simulink library "Lib_Piccolo"  (R2018b)
settings: Solver=VariableStepAuto  StartTime=0.0  StopTime=10.0  RelTol=1e-3
values from neighbouring files (symbols this model uses):
  AccelErrInt2Brakes = 0.15    [SimulationControlConfig16P.m]    (also in SimulationControlConfig16P_F0.m; SimulationControlConfig16P_F2.m; SimulationControlConfig16P_LEGACY.m; SimulationControlConfigTAILLESS.m = 0.2)
  AileronMax = 25    [SimulationControlConfig16P.m]    (also in SimulationControlConfig16P_F0.m; SimulationControlConfig16P_F2.m; SimulationControlConfig16P_LEGACY.m; SimulationControlConfigTAILLESS.m)
  AileronPower = 0.00268    [SimulationControlConfig16P.m]    (also in SimulationControlConfig16P_F0.m; SimulationControlConfig16P_F2.m; SimulationControlConfig16P_LEGACY.m; SimulationControlConfigTAILLESS.m = 0.002266)
  AileronSurfaceMax = 45    [SimulationControlConfig16P.m]    (also in SimulationControlConfig16P_F0.m; SimulationControlConfig16P_F2.m; SimulationControlConfig16P_LEGACY.m; SimulationControlConfigTAILLESS_CGAFT_F0.m = 25)
  AileronTrim = 0    [SimulationControlConfig16P.m]    (also in SimulationControlConfig16P_F0.m; SimulationControlConfig16P_F2.m; SimulationControlConfig16P_LEGACY.m; SimulationControlConfigTAILLESS.m)
  Alt = 1000 + TerrainHeight    [SimulationStateConfig.m]
  AltCruise_m = Alt * 0.3048    [SimulationControlConfig16P.m]    (also in SimulationControlConfig16P_F2.m; SimulationControlConfigTAILLESS.m = Alt/3.28084; SimulationControlConfigTAILLESS_CGAFT_F0.m = 640; SimulationControlConfigTAILLESS_CGFWD_F0.m = 640)
  AltitudeRate2PitchCmdIntegratorInit = 0.1    [SimulationControlPre.m]
  AltMax = 10000    [SimulationControlConfig16P.m]    (also in SimulationControlConfig16P_F0.m; SimulationControlConfig16P_F2.m; SimulationControlConfig16P_LEGACY.m; SimulationControlConfigTAILLESS.m)
  AltMaxAccel = 2.5    [SimulationControlConfig16P.m]    (also in SimulationControlConfig16P_F0.m = 2; SimulationControlConfig16P_F2.m = 2; SimulationControlConfig16P_LEGACY.m = 0.9; SimulationControlConfigTAILLESS.m = 2)
  AltMin = 0    [SimulationControlConfig16P.m]    (also in SimulationControlConfig16P_F0.m; SimulationControlConfig16P_F2.m; SimulationControlConfig16P_LEGACY.m; SimulationControlConfigTAILLESS.m)
  AltRateCmd2Pitch = 0.26    [SimulationControlConfig16P.m]    (also in SimulationControlConfig16P_F0.m = 0.35; SimulationControlConfig16P_F2.m = 0.35; SimulationControlConfig16P_LEGACY.m = 0.6; SimulationControlConfigTAILLESS.m = 0.9)
  AltRateError2Pitch = 0.34    [SimulationControlConfig16P.m]    (also in SimulationControlConfig16P_F0.m = 0.61; SimulationControlConfig16P_F2.m = 0.61; SimulationControlConfig16P_LEGACY.m = 0.4; SimulationControlConfigTAILLESS.m = 0.3)
  AltRateErrorInt2Pitch = 0.61    [SimulationControlConfig16P.m]    (also in SimulationControlConfig16P_F0.m = 0.28; SimulationControlConfig16P_F2.m = 0.28; SimulationControlConfig16P_LEGACY.m = 0.45; SimulationControlConfigTAILLESS.m = 0.15)
  AltRateLpfCutOff = 3    [SimulationControlConfig16P.m]    (also in SimulationControlConfig16P_F0.m; SimulationControlConfig16P_F2.m; SimulationControlConfig16P_LEGACY.m; SimulationControlConfigTAILLESS.m = 5)
  AutoNosegear2Rudder = 26    [SimulationControlConfig16P.m]    (also in SimulationControlConfig16P_F0.m; SimulationControlConfig16P_F2.m; SimulationControlConfig16P_LEGACY.m; SimulationControlConfigTAILLESS.m = 25.2)
  b = 5.54    [SimulationControlConfig16P.m]    (also in SimulationControlConfig16P_F0.m; SimulationControlConfig16P_F2.m; SimulationControlConfig16P_LEGACY.m; SimulationControlConfigTAILLESS.m = 2.37)
  Bank2AileronIntegratorInit = 0    [SimulationControlPre.m]
  BankMax_User = BankMax_User/180*pi    (= 0.610865238198)    [SimulationControlConfig16P.m]    (also in SimulationControlConfig16P_F0.m = 0.523598775598; SimulationControlConfig16P_F2.m = 0.523598775598; SimulationControlConfig16P_LEGACY.m = 0.523598775598; SimulationControlConfigTAILLESS.m = 0.558505360638)
  baseLegFlaps = 20    [SimulationControlConfig16P.m]    (also in SimulationControlConfig16P_F0.m; SimulationControlConfig16P_F2.m = 15; SimulationControlConfig16P_LEGACY.m = 0; SimulationControlConfigTAILLESS.m = 0)
  C = GeneticOpt.C    [SimulationCostFunction.m]
  c = Sw/b    (= 0.841696750903)    [SimulationControlConfig16P.m]    (also in SimulationControlConfig16P_F0.m; SimulationControlConfig16P_F2.m; SimulationControlConfig16P_LEGACY.m; SimulationControlConfigTAILLESS.m = 0.354008438819)
  cell2WheelFactorMG = 5.98    [SimulationSensorConfig16P_LEGACY.m]
  cell2WheelFactorNG = 1    [SimulationSensorConfig16P_LEGACY.m]
  cellSatMaxMG = 15000    [SimulationSensorConfig16P.m]    (also in SimulationSensorConfig16P_LEGACY.m; SimulationSensorConfigTAILLESS7P.m; SimulationSensorConfigUTAIL7P.m)
  cellSatMaxNG = 1000    [SimulationSensorConfig16P.m]    (also in SimulationSensorConfig16P_LEGACY.m; SimulationSensorConfigTAILLESS7P.m; SimulationSensorConfigUTAIL7P.m)
  cellSatMinMG = -15000    [SimulationSensorConfig16P.m]    (also in SimulationSensorConfig16P_LEGACY.m; SimulationSensorConfigTAILLESS7P.m; SimulationSensorConfigUTAIL7P.m)
  cellSatMinNG = -1000    [SimulationSensorConfig16P.m]    (also in SimulationSensorConfig16P_LEGACY.m; SimulationSensorConfigTAILLESS7P.m; SimulationSensorConfigUTAIL7P.m)
  CL_Limit = CL_Max    (= 0.54)    [SimulationControlConfig16P.m]    (also in SimulationControlConfig16P_F0.m; SimulationControlConfig16P_F2.m = 0.638; SimulationControlConfig16P_LEGACY.m; SimulationControlConfigTAILLESS.m = 0.525)
  CL_Max = 0.54    [SimulationControlConfig16P.m]    (also in SimulationControlConfig16P_F0.m; SimulationControlConfig16P_F2.m = 0.638; SimulationControlConfig16P_LEGACY.m; SimulationControlConfigTAILLESS.m = 0.525)
  CL_Max_Nom = 0.465    [SimulationControlConfig16P.m]    (also in SimulationControlConfig16P_F0.m; SimulationControlConfig16P_F2.m = 0.563; SimulationControlConfig16P_LEGACY.m; SimulationControlConfigTAILLESS.m = 0.39)
  CL_Min = 0    [SimulationControlConfig16P.m]    (also in SimulationControlConfig16P_F0.m; SimulationControlConfig16P_F2.m; SimulationControlConfig16P_LEGACY.m; SimulationControlConfigTAILLESS.m)
  ClimbMaxFraction = 0.35    [SimulationControlConfig16P.m]    (also in SimulationControlConfig16P_F0.m = 0.17; SimulationControlConfig16P_F2.m = 0.17; SimulationControlConfig16P_LEGACY.m = 0.24; SimulationControlConfigTAILLESS.m = 0.21)
  ClimboutMaxBank = 7.0    (= 7)    [SimulationControlConfig16P.m]    (also in SimulationControlConfig16P_F0.m; SimulationControlConfig16P_F2.m; SimulationControlConfig16P_LEGACY.m; SimulationControlConfigTAILLESS.m = 5)
  ClimboutTimer = 7.0    (= 7)    [SimulationControlConfig16P.m]    (also in SimulationControlConfig16P_F0.m; SimulationControlConfig16P_F2.m; SimulationControlConfig16P_LEGACY.m; SimulationControlConfigTAILLESS.m)
  dCl_per_dFlap = 0.005581818    [SimulationControlConfig16P.m]    (also in SimulationControlConfig16P_F0.m = 0; SimulationControlConfig16P_F2.m = 0.0065; SimulationControlConfig16P_LEGACY.m = 0; SimulationControlConfigTAILLESS.m = 0)
  DecelerationCmd = 3.1    [SimulationControlConfig16P.m]    (also in SimulationControlConfig16P_F0.m; SimulationControlConfig16P_F2.m; SimulationControlConfig16P_LEGACY.m; SimulationControlConfigTAILLESS.m = 0.1)
  DeRotateLogicEndTimer = abs((NoseDownLimit_Deg-1)/DeRotateRamp_Dps)    [SimulationControlConfig16P.m]    (also in SimulationControlConfig16P_F0.m; SimulationControlConfig16P_F2.m; SimulationControlConfig16P_LEGACY.m; SimulationControlConfigTAILLESS.m)
  DeRotateLogicHoldNoseUpTimer = 0.1    [SimulationControlConfig16P.m]    (also in SimulationControlConfig16P_F0.m; SimulationControlConfig16P_F2.m; SimulationControlConfig16P_LEGACY.m; SimulationControlConfigTAILLESS.m)
  DeRotateLogicTimerTimeout = 2    [SimulationControlConfig16P.m]    (also in SimulationControlConfig16P_F0.m; SimulationControlConfig16P_F2.m; SimulationControlConfig16P_LEGACY.m; SimulationControlConfigTAILLESS.m)
  DeRotateLowerCmdSaturation = 0    [SimulationControlConfig16P.m]    (also in SimulationControlConfig16P_F0.m; SimulationControlConfig16P_F2.m; SimulationControlConfig16P_LEGACY.m; SimulationControlConfigTAILLESS.m)
  DeRotateRamp_Dps = 3    [SimulationControlConfig16P.m]    (also in SimulationControlConfig16P_F0.m; SimulationControlConfig16P_F2.m; SimulationControlConfig16P_LEGACY.m; SimulationControlConfigTAILLESS.m = 8)
  DeRotateUpperCmdSaturation = 7    [SimulationControlConfig16P.m]    (also in SimulationControlConfig16P_F0.m; SimulationControlConfig16P_F2.m; SimulationControlConfig16P_LEGACY.m; SimulationControlConfigTAILLESS.m)
  DescentMaxFraction = 0.22    [SimulationControlConfig16P.m]    (also in SimulationControlConfig16P_F0.m = 0.2; SimulationControlConfig16P_F2.m = 0.2; SimulationControlConfig16P_LEGACY.m = 0.2; SimulationControlConfigTAILLESS.m = 0.17)
  DesktopSimTerrainOffset_m = 0.406    [SimulationAircraftConfig.m]
  downwindFlaps = 0    [SimulationControlConfig16P.m]    (also in SimulationControlConfig16P_F0.m; SimulationControlConfig16P_F2.m = 15; SimulationControlConfig16P_LEGACY.m; SimulationControlConfigTAILLESS.m)
  downwindSplitAil = 0    [SimulationControlConfig16P_F2.m]
  DP_init = 0.5*1.225*V_init^2    [SimulationControlConfig16P.m]    (also in SimulationControlConfig16P_F0.m; SimulationControlConfig16P_F2.m; SimulationControlConfig16P_LEGACY.m; SimulationControlConfigTAILLESS.m)
  dscNoiseMG = 1    [SimulationSensorConfig16P_LEGACY.m]
  dscNoiseNG = 0.25    [SimulationSensorConfig16P_LEGACY.m]
  DSCnumBits = 24    [SimulationSensorConfig16P.m]    (also in SimulationSensorConfig16P_LEGACY.m; SimulationSensorConfigTAILLESS7P.m; SimulationSensorConfigUTAIL7P.m)
  DSCRangeMaxMG = 15000    [SimulationSensorConfig16P.m]    (also in SimulationSensorConfig16P_LEGACY.m; SimulationSensorConfigTAILLESS7P.m; SimulationSensorConfigUTAIL7P.m)
  DSCRangeMaxNG = 1000    [SimulationSensorConfig16P.m]    (also in SimulationSensorConfig16P_LEGACY.m; SimulationSensorConfigTAILLESS7P.m; SimulationSensorConfigUTAIL7P.m)
  DSCRangeMinMG = -15000    [SimulationSensorConfig16P.m]    (also in SimulationSensorConfig16P_LEGACY.m; SimulationSensorConfigTAILLESS7P.m; SimulationSensorConfigUTAIL7P.m)
  DSCRangeMinNG = -1000    [SimulationSensorConfig16P.m]    (also in SimulationSensorConfig16P_LEGACY.m; SimulationSensorConfigTAILLESS7P.m; SimulationSensorConfigUTAIL7P.m)
  dt = DLLSim.dt    [SimulationTimeStep.m]    (also in SimulationTrim.m = 0.02)
  EarlyTouchdownThreshold = 3.0    (= 3)    [SimulationControlConfig16P.m]    (also in SimulationControlConfig16P_F0.m; SimulationControlConfig16P_F2.m; SimulationControlConfig16P_LEGACY.m; SimulationControlConfigTAILLESS.m)
  ElevatorDeflectionRate = 15    [SimulationControlConfig16P.m]    (also in SimulationControlConfig16P_F0.m; SimulationControlConfig16P_F2.m; SimulationControlConfig16P_LEGACY.m = 12; SimulationControlConfigTAILLESS.m = 5)
  ElevatorMax = 25    [SimulationControlConfig16P.m]    (also in SimulationControlConfig16P_F0.m; SimulationControlConfig16P_F2.m; SimulationControlConfig16P_LEGACY.m; SimulationControlConfigTAILLESS.m)
  ElevatorPower = -0.002209    [SimulationControlConfig16P.m]    (also in SimulationControlConfig16P_F0.m; SimulationControlConfig16P_F2.m; SimulationControlConfig16P_LEGACY.m; SimulationControlConfigTAILLESS.m = -0.002668)
  ElevatorTrim = -3.5    [SimulationControlConfig16P.m]    (also in SimulationControlConfig16P_F0.m; SimulationControlConfig16P_F2.m; SimulationControlConfig16P_LEGACY.m; SimulationControlConfigTAILLESS.m = -3)
  elevonBias = 0    [SimulationControlConfig16P.m]    (also in SimulationControlConfig16P_F0.m; SimulationControlConfig16P_F2.m; SimulationControlConfig16P_LEGACY.m; SimulationControlConfigTAILLESS.m)
  Enable_TAS_Protection = 0    [SimulationControlConfig16P.m]    (also in SimulationControlConfig16P_F0.m; SimulationControlConfig16P_F2.m; SimulationControlConfig16P_LEGACY.m; SimulationControlConfigTAILLESS.m)
  EnableCrossTrackAbort = 1    [SimulationControlConfig16P.m]    (also in SimulationControlConfigTAILLESS.m; SimulationControlConfigTAILLESS_CGAFT_F0.m; SimulationControlConfigTAILLESS_CGFWD_F0.m; SimulationControlConfigTAILLESS_CGFWD_F2.m)
  EnergyBandwidth = 0.04    [SimulationControlConfig16P.m]    (also in SimulationControlConfig16P_F0.m = 0.03; SimulationControlConfig16P_F2.m = 0.03; SimulationControlConfig16P_LEGACY.m = 0.02; SimulationControlConfigTAILLESS.m = 0.06)
  EngineLhFuelCut = 0    [SimulationAircraftConfig.m]
  EngineRhFuelCut = 0    [SimulationAircraftConfig.m]
  FastThrottleRate = 0.075    [SimulationControlConfig16P.m]    (also in SimulationControlConfig16P_F0.m = 0.05; SimulationControlConfig16P_F2.m = 0.05; SimulationControlConfig16P_LEGACY.m = 0.05; SimulationControlConfigTAILLESS.m = 0.1)
  FilterWarmUpTime = 2    [SimulationSensorConfig16P.m]    (also in SimulationSensorConfig16P_LEGACY.m; SimulationSensorConfigTAILLESS7P.m; SimulationSensorConfigUTAIL7P.m)
  finalApproachFlaps = 20    [SimulationControlConfig16P.m]    (also in SimulationControlConfig16P_F0.m; SimulationControlConfig16P_F2.m = 15; SimulationControlConfig16P_LEGACY.m = 0; SimulationControlConfigTAILLESS.m = 0)
  finalApproachSplitAil = 20    [SimulationControlConfig16P_F2.m]
  FinalDescentSlope_Deg = testPlans(testIndx).descentSlope    [SimulationControlConfig16P.m]    (also in SimulationControlConfig16P_F0.m; SimulationControlConfig16P_F2.m; SimulationControlConfig16P_LEGACY.m; SimulationControlConfigTAILLESS.m)
  flapMax = 0    [SimulationControlConfig16P.m]    (also in SimulationControlConfig16P_F0.m = 35; SimulationControlConfig16P_F2.m = 33; SimulationControlConfig16P_LEGACY.m; SimulationControlConfigTAILLESS.m)
  flapRate = 7.5    [SimulationControlConfig16P.m]    (also in SimulationControlConfig16P_F0.m; SimulationControlConfig16P_F2.m; SimulationControlConfig16P_LEGACY.m; SimulationControlConfigTAILLESS.m = 6.6)
  FlareHeight = 5    [SimulationControlConfig16P.m]    (also in SimulationControlConfig16P_F0.m; SimulationControlConfig16P_F2.m; SimulationControlConfig16P_LEGACY.m = 4.8; SimulationControlConfigTAILLESS.m = 2.75)
  FlareVerticalRate_mps = -0.4    [SimulationControlConfig16P.m]    (also in SimulationControlConfig16P_F0.m; SimulationControlConfig16P_F2.m; SimulationControlConfig16P_LEGACY.m = -0.5; SimulationControlConfigTAILLESS.m = -0.15)
  Fp_Aileron = 0.55*2*pi*RollRateLpfCutoff*dt    [SimulationControlConfig16P.m]    (also in SimulationControlConfig16P_F0.m; SimulationControlConfig16P_F2.m; SimulationControlConfig16P_LEGACY.m; SimulationControlConfigTAILLESS.m)
  Fp_Alt = 2*pi*0.55*AltBandwidth    (= 0.622035345411)    [SimulationControlConfig16P.m]    (also in SimulationControlConfig16P_F0.m; SimulationControlConfig16P_F2.m; SimulationControlConfig16P_LEGACY.m = 0.099; SimulationControlConfigTAILLESS.m = 0.207345115137)
  Fp_AltRate = 0.55*2*pi*AltRateLpfCutOff*dt    [SimulationControlConfig16P.m]    (also in SimulationControlConfig16P_F0.m; SimulationControlConfig16P_F2.m; SimulationControlConfig16P_LEGACY.m; SimulationControlConfigTAILLESS.m)
  Fp_Elevator = 0.55*2*pi*PitchRateLpfCutoff*dt    [SimulationControlConfig16P.m]    (also in SimulationControlConfig16P_F0.m; SimulationControlConfig16P_F2.m; SimulationControlConfig16P_LEGACY.m; SimulationControlConfigTAILLESS.m)
  Fp_Energy = 0.55*2*pi*EnergyBandwidth    (= 0.138230076758)    [SimulationControlConfig16P.m]    (also in SimulationControlConfig16P_F0.m = 0.103672557568; SimulationControlConfig16P_F2.m = 0.103672557568; SimulationControlConfig16P_LEGACY.m = 0.069115038379; SimulationControlConfigTAILLESS.m = 0.207345115137)
  Fp_Energy2 = 0.55*2*pi*EnergyBandwidth*dt    [SimulationControlConfig16P.m]    (also in SimulationControlConfig16P_F0.m; SimulationControlConfig16P_F2.m; SimulationControlConfig16P_LEGACY.m; SimulationControlConfigTAILLESS.m)
  Fp_Pitch = 0.55*2*pi*PitchBandwidth    (= 2.45358386245)    [SimulationControlConfig16P.m]    (also in SimulationControlConfig16P_F0.m; SimulationControlConfig16P_F2.m = 1.72787595947; SimulationControlConfig16P_LEGACY.m = 3.11017672705; SimulationControlConfigTAILLESS.m = 1.55508836353)
  Fp_Pitch_2 = 0.55*2*pi*PitchBandwidth*dt    [SimulationControlConfig16P.m]    (also in SimulationControlConfig16P_F0.m; SimulationControlConfig16P_F2.m; SimulationControlConfig16P_LEGACY.m; SimulationControlConfigTAILLESS.m)
  Fp_Roll = RollBandwidth^2    (= 1.69)    [SimulationControlConfig16P.m]    (also in SimulationControlConfig16P_F0.m = 1.44; SimulationControlConfig16P_F2.m = 1.44; SimulationControlConfig16P_LEGACY.m = 1.44; SimulationControlConfigTAILLESS.m = 1.21)
  Fp_Rudder = 0.55*2*pi*YawRateLpfCutoff*dt    [SimulationControlConfig16P.m]    (also in SimulationControlConfig16P_F0.m; SimulationControlConfig16P_F2.m; SimulationControlConfig16P_LEGACY.m; SimulationControlConfigTAILLESS.m)
  Fp_TAS = 0.55*2*pi*TASBandwidth    (= 0.103672557568)    [SimulationControlConfig16P.m]    (also in SimulationControlConfig16P_F0.m; SimulationControlConfig16P_F2.m; SimulationControlConfig16P_LEGACY.m; SimulationControlConfigTAILLESS.m = 0.172787595947)
  Fp_TAS_Filter = 2*pi*TasLpfCutoff*dt    [SimulationControlConfig16P.m]    (also in SimulationControlConfig16P_F0.m; SimulationControlConfig16P_F2.m; SimulationControlConfig16P_LEGACY.m; SimulationControlConfigTAILLESS.m)
  Fp_Turn = 0.55*2*pi*TurnErrLPFcutoff    (= 0.172787595947)    [SimulationControlConfig16P.m]    (also in SimulationControlConfig16P_F0.m = 0.0345575191895; SimulationControlConfig16P_F2.m = 0.0345575191895; SimulationControlConfig16P_LEGACY.m = 0.0345575191895; SimulationControlConfigTAILLESS.m)
  Fp_TurnDerr = 0.55*2*pi*TurnDerivativeLPFcutoff    (= 0.172787595947)    [SimulationControlConfig16P.m]    (also in SimulationControlConfig16P_F0.m = 0.0345575191895; SimulationControlConfig16P_F2.m = 0.0345575191895; SimulationControlConfig16P_LEGACY.m = 0.0345575191895; SimulationControlConfigTAILLESS.m)
  FTV = 3    [SimulationAircraftConfig.m]
  ftvStaticPositionError = 1/1.18    (= 0.847457627119)    [SimulationSensorConfig16P.m]    (also in SimulationSensorConfig16P_LEGACY.m; SimulationSensorConfigTAILLESS7P.m = 1; SimulationSensorConfigUTAIL7P.m = 1)
  g = 9.81    [SimulationStateConfig.m]
  goAroundSplitAil = 0    [SimulationControlConfig16P_F2.m]
  GustSpd_Kts = testPlans(testIndx).gustSpd    [SimulationStateConfig.m]
  GustTriggerVal = testPlans(testIndx).gustTriggerVal    [SimulationStateConfig.m]
  HeadingErr2TurnRate = 0.5    [SimulationControlConfig16P.m]    (also in SimulationControlConfig16P_F0.m; SimulationControlConfig16P_F2.m; SimulationControlConfig16P_LEGACY.m; SimulationControlConfigTAILLESS.m)
  HeadingErrDer2TurnRate = 0.3    [SimulationControlConfig16P.m]    (also in SimulationControlConfig16P_F0.m; SimulationControlConfig16P_F2.m; SimulationControlConfig16P_LEGACY.m; SimulationControlConfigTAILLESS.m)
  IASbounce = IASstall*0.8    [SimulationControlPre.m]
  IAScruiseCMD = sqrt(2*m*9.81/(1.225*Sw*CL_cruise))    [SimulationControlConfig16P.m]    (also in SimulationControlConfig16P_F0.m; SimulationControlConfig16P_F2.m; SimulationControlConfig16P_LEGACY.m; SimulationControlConfigTAILLESS.m)
  IASfinalCMD = 1.12 * IASmin    [SimulationControlConfig16P.m]    (also in SimulationControlConfig16P_F0.m = 1.14 * IASmin; SimulationControlConfig16P_F2.m = 1.10 * IASmin; SimulationControlConfig16P_LEGACY.m = 1.10 * IASmin; SimulationControlConfigTAILLESS.m = 1.14 * IASmin)
  IASflareCMD = IASstall    [SimulationControlConfig16P.m]    (also in SimulationControlConfig16P_F0.m; SimulationControlConfig16P_F2.m; SimulationControlConfig16P_LEGACY.m; SimulationControlConfigTAILLESS.m)
  IASmax = 64    [SimulationControlConfig16P.m]    (also in SimulationControlConfig16P_F0.m = 46; SimulationControlConfig16P_F2.m = 52; SimulationControlConfig16P_LEGACY.m = 46; SimulationControlConfigTAILLESS.m = 38.9)
  IASmin = sqrt(2*m*9.81/(1.225*Sw*0.9*CL_Max_Nom))    [SimulationControlConfig16P.m]    (also in SimulationControlConfig16P_F0.m; SimulationControlConfig16P_F2.m; SimulationControlConfig16P_LEGACY.m; SimulationControlConfigTAILLESS.m)
  IASshortCMD = IASstall    [SimulationControlConfig16P.m]    (also in SimulationControlConfig16P_F0.m; SimulationControlConfig16P_F2.m; SimulationControlConfig16P_LEGACY.m; SimulationControlConfigTAILLESS.m)
  IASstall = sqrt(2*m*9.81/(1.225*Sw*CL_Max))    [SimulationControlConfig16P.m]    (also in SimulationControlConfig16P_F0.m; SimulationControlConfig16P_F2.m; SimulationControlConfig16P_LEGACY.m; SimulationControlConfigTAILLESS.m)
  inFlight = 1    [SimulationControlConfig16P.m]    (also in SimulationControlConfigTAILLESS.m; SimulationControlConfigTAILLESS_CGAFT_F0.m; SimulationControlConfigTAILLESS_CGFWD_F0.m; SimulationControlConfigTAILLESS_CGFWD_F2.m)
  JetCatOffset = 5    [SimulationControlConfig16P.m]    (also in SimulationControlConfig16P_F0.m; SimulationControlConfig16P_F2.m; SimulationControlConfig16P_LEGACY.m)
  LaunchRollingElevator = -1.5    [SimulationControlConfig16P.m]    (also in SimulationControlConfig16P_F0.m; SimulationControlConfig16P_F2.m = 1.25; SimulationControlConfig16P_LEGACY.m; SimulationControlConfigTAILLESS.m = 1)
  ldg_NosegearMax = 10    [SimulationControlConfig16P.m]    (also in SimulationControlConfig16P_F0.m; SimulationControlConfig16P_F2.m; SimulationControlConfig16P_LEGACY.m; SimulationControlConfigTAILLESS.m)
  ldg_TrackVyErrInt2Nosegear = 0.1250    (= 0.125)    [SimulationControlConfig16P.m]    (also in SimulationControlConfig16P_F0.m; SimulationControlConfig16P_F2.m; SimulationControlConfig16P_LEGACY.m; SimulationControlConfigTAILLESS.m = 0.00714285714286)
  ldg_TrackVyErrPro2Nosegear = 0.35    [SimulationControlConfig16P.m]    (also in SimulationControlConfig16P_F0.m; SimulationControlConfig16P_F2.m; SimulationControlConfig16P_LEGACY.m; SimulationControlConfigTAILLESS.m = 0.0546666666667)
  ldg_TrackY2Vy = 0.07    [SimulationControlConfig16P.m]    (also in SimulationControlConfig16P_F0.m; SimulationControlConfig16P_F2.m; SimulationControlConfig16P_LEGACY.m; SimulationControlConfigTAILLESS.m = 0.17)
  ldg_Vy2NosegearScalingPower = 1.075    [SimulationControlConfig16P.m]    (also in SimulationControlConfig16P_F0.m; SimulationControlConfig16P_F2.m; SimulationControlConfig16P_LEGACY.m; SimulationControlConfigTAILLESS.m = 0.6)
  ldg_Y2VyScalingPower = 0.175    [SimulationControlConfig16P.m]    (also in SimulationControlConfig16P_F0.m; SimulationControlConfig16P_F2.m; SimulationControlConfig16P_LEGACY.m; SimulationControlConfigTAILLESS.m = 0)
  ldg_YawRate2Nosegear = 0.175    [SimulationControlConfig16P.m]    (also in SimulationControlConfig16P_F0.m; SimulationControlConfig16P_F2.m; SimulationControlConfig16P_LEGACY.m; SimulationControlConfigTAILLESS.m = 0.065)
  LiftSlope = 0.064285    [SimulationControlConfig16P.m]    (also in SimulationControlConfig16P_F0.m; SimulationControlConfig16P_F2.m; SimulationControlConfig16P_LEGACY.m; SimulationControlConfigTAILLESS.m = 0.058631)
  LPFaileronInit = 0    [SimulationControlPre.m]
  LPFclestInit = 0    [SimulationControlPre.m]
  LPFenergyFFInit = 0    [SimulationControlPre.m]
  ... (+122 more)
undefined symbols (not defined in the file or in its folder): abortFlag, alphaHPF, apmDelay, BRWNOUT, CRAWOR, CRAWUR, DiscIntNeverNeededParam, DLLSim, DLLSimStep, ECOMOR, ECOMUR, Fp_Tas, GustTrigger_HeightAgl_m, IPSTAT, LCINTEG, Ldg_Persist_Time, LOWER_FLAGS, MSG_ENABLE, NoiseStd, OLDVAL, OVERRIDE_ENABLE, OVERRIDE_VALUE, REBOOT, reversionEnable, revIASMax, revIASMin, revPitchMax, revPitchMin, revPitchRateMax, revRollMax, revRollRateMax, SAMPLE, SCALON, SensorModel, sigbuilder_block, Sim_Vx, Sim_Vy, Sim_Vz, Sim_Xpos, Sim_Ypos, Sim_Zpos, SYSOR, SYSUR, TARE, TEMPOR, TEMPUR, testIndx, testPlan, testPlans, Trim_piccoloInCmd, Trim_REFSI_FD_IN_nmodeCgShifterCmd_Flag, Trim_REFSI_FD_IN_nmodeCgShifterCmd_Ft, Trim_REFSI_FD_IN_nmodeCgShifterCmdType, Trim_REFSI_FD_IN_nmodeCgShifterNRCActive, Trim_REFSI_FD_IN_nmodeFlapLhIBCmd_Deg, Trim_REFSI_FD_IN_nmodeFlapLhOBCmd_Deg, Trim_REFSI_FD_IN_nmodeFlapRhIBCmd_Deg, Trim_REFSI_FD_IN_nmodeFlapRhOBCmd_Deg, Trim_REFSI_FD_IN_nmodeSlatLhCmd_Deg ... (+11)
libraries: simulink x1237, $bdroot x179, aerolibconvert2 x63, dspswit3 x25, aerolibatmos2 x5, simulink_extras x4, dsparch4 x2, Lib_Piccolo_Alt x2, eeGeneralControl x1, dspindex x1
(part 13 of 74)

== system Lib_Piccolo/DSC Load Conversion/DSC-to-Wheel MGL ==
  DSC_Load_N : Inport
  DSC-to-Wheel Global Linear Scaling : Subsystem
  DSC-to-Wheel Polynomial Scaling MGL : Subsystem
  Switch : Switch  Criteria=u2 > Threshold  Threshold=SensorModel.WOW.Cell.intercept.MGL  OutDataTypeStr=single
  MGL_WOW_N : Outport  VectorParamsAs1DForOutWhenUnconnected=on
  wires:
  DSC_Load_N/1 -> DSC-to-Wheel Global Linear Scaling/1(DSC_Load_N), DSC-to-Wheel Polynomial Scaling MGL/1(DSC_Load_N), Switch/2
  DSC-to-Wheel Global Linear Scaling/1(WOW_N) -> Switch/1
  Switch/1 -> MGL_WOW_N/1
  DSC-to-Wheel Polynomial Scaling MGL/1(WOW_N) -> Switch/3

== system Lib_Piccolo/DSC Load Conversion/DSC-to-Wheel MGR ==
  DSC_Load_N : Inport
  DSC-to-Wheel Global Linear Scaling : Subsystem
  DSC-to-Wheel Polynomial Scaling MGR : Subsystem
  Switch : Switch  Criteria=u2 > Threshold  Threshold=SensorModel.WOW.Cell.intercept.MGR  OutDataTypeStr=single
  MGR_WOW_N : Outport  OutDataTypeStr=single  VectorParamsAs1DForOutWhenUnconnected=on
  wires:
  DSC_Load_N/1 -> Switch/2, DSC-to-Wheel Polynomial Scaling MGR/1(DSC_Load_N), DSC-to-Wheel Global Linear Scaling/1(DSC_Load_N)
  DSC-to-Wheel Polynomial Scaling MGR/1(WOW_N) -> Switch/3
  Switch/1 -> MGR_WOW_N/1
  DSC-to-Wheel Global Linear Scaling/1(WOW_N) -> Switch/1

== system Lib_Piccolo/DSC Load Conversion/DSC-to-Wheel NG ==
  DSC_Load_N : Inport
  DSC-to-Wheel Polynomial Scaling NG : Subsystem
  NG_WOW_N : Outport  OutDataTypeStr=single  VectorParamsAs1DForOutWhenUnconnected=on
  wires:
  DSC-to-Wheel Polynomial Scaling NG/1(WOW_N) -> NG_WOW_N/1
  DSC_Load_N/1 -> DSC-to-Wheel Polynomial Scaling NG/1(DSC_Load_N)

== system Lib_Piccolo/Emulated INS/Accelerometer Noise Model ==
  XAccel_mps2 : Inport
  Yaccel_mps2 : Inport  Port=2
  Zaccel_mps2 : Inport  Port=3
  Bus Element In2 : Inport  Port=4  PortName=contactBus  Element=GrndContactRMG
  Bus Element In : Inport  Port=4  PortName=contactBus  Element=GrndContactNG
  Bus Element In1 : Inport  Port=4  PortName=contactBus  Element=GrndContactLMG
  gndSpeed_mps : Inport  Port=5
  Generate Accel Noise : Subsystem
  OR : Logic  Operator=OR  Inputs=3  IconShape=distinctive  AllPortsSameDT=off  OutDataTypeStr=boolean
  Saturation : Saturate  UpperLimit=98  LowerLimit=-98
  Saturation1 : Saturate  UpperLimit=98  LowerLimit=-98
  Saturation2 : Saturate  UpperLimit=98  LowerLimit=-98
  Sum : Sum  Inputs=|++
  Sum1 : Sum  Inputs=|++
  Sum2 : Sum  Inputs=|++
  xAccel_mps2 : Outport
  yAccel_mps : Outport  Port=2
  zAccel_mps : Outport  Port=3
  wires:
  gndSpeed_mps/1 -> Generate Accel Noise/2(gndSpeed_mps)
  Generate Accel Noise/3(NoiseZaccelmps2) -> Sum2/2
  Generate Accel Noise/2(NoiseYaccelmps2) -> Sum1/2
  Generate Accel Noise/1(NoiseXaccelmps2) -> Sum/2
  OR/1 -> Generate Accel Noise/1(ContactBool)
  Bus Element In1/1 -> OR/2
  Bus Element In/1 -> OR/1
  Bus Element In2/1 -> OR/3
  Saturation1/1 -> yAccel_mps/1  "Yaccel_mps2"
  Saturation/1 -> xAccel_mps2/1  "XAccel_mps2"
  Saturation2/1 -> zAccel_mps/1  "Zaccel_mps2"
  XAccel_mps2/1 -> Sum/1
  Yaccel_mps2/1 -> Sum1/1
  Zaccel_mps2/1 -> Sum2/1
  Sum2/1 -> Saturation2/1  "Zaccel_mps2"
  Sum1/1 -> Saturation1/1  "Yaccel_mps2"
  Sum/1 -> Saturation/1  "XAccel_mps2"

== system Lib_Piccolo/Emulated INS LEGACY/LPF TAS ==
  Input : Inport
  Reset : Inport  Port=2
  Add1 : Sum  Inputs=++|
  Compare To Constant2 : simulink/Logic and Bit Operations/Compare To Constant  relop=>  const=0  OutDataTypeStr=uint8
  Constant11 : Constant  Value=TasLpfCutoff
  Switch1 : Switch  Criteria=u2 > Threshold
  Unit Delay1 : UnitDelay  InitialCondition=LPFtasInit  SampleTime=-1
  a1 : Gain  Gain=1-Fp_Tas
  b0 : Gain  Gain=Fp_Tas
  Output : Outport
  wires:
  Constant11/1 -> Compare To Constant2/1
  Compare To Constant2/1 -> Switch1/2
  Switch1/1 -> Output/1
  Input/1 -> b0/1, Switch1/3
  Add1/1 -> Switch1/1, Unit Delay1/1
  a1/1 -> Add1/1
  b0/1 -> Add1/2
  Unit Delay1/1 -> a1/1

== system Lib_Piccolo/Ground Detection Systems/CL Detection Wrapper ==
  note: -1 indicates disarmed. Reverts to using CL touchdown detection
  WoWarmed : Inport
  FeedbackBus : Inport  Port=2
  AND : Logic  IconShape=distinctive  AllPortsSameDT=off  OutDataTypeStr=boolean
  Bus Selector : BusSelector  OutputSignals=apMode,zAccel_Body_mps2,DynamicPressure_Pa
  CL Based Touchdown Detection Logic : Subsystem
  Compare To Constant1 : simulink/Logic and Bit Operations/Compare To Constant  relop=>=  const=9  OutDataTypeStr=uint8
  Divide : Product  Inputs=*/
  Extended Range : Saturate  UpperLimit=2  LowerLimit=-2
  Gain : Gain  Gain=m/Sw
  OR : Logic  Operator=OR  IconShape=distinctive  AllPortsSameDT=off  OutDataTypeStr=boolean
  Terminator : Terminator
  Terminator1 : Terminator
  TouchdownDetected : Outport
  tag scope: Sim_CLdetect_Signal=global, Sim_CLest=global
  wires:
  OR/1 -> AND/1
  WoWarmed/1 -> CL Based Touchdown Detection Logic/1(Pic_WOW)
  Compare To Constant1/1 -> AND/2
  Extended Range/1 -> [Sim_CLest], CL Based Touchdown Detection Logic/3(CL)  "Sim.CLest"
  Gain/1 -> Divide/1
  Bus Selector/1 -> Compare To Constant1/1, CL Based Touchdown Detection Logic/2(Pic_APMode)  "<apMode>"
  Divide/1 -> Extended Range/1
  AND/1 -> [Sim_CLdetect_Signal], TouchdownDetected/1  "Sim_CLdetect_Signal"
  CL Based Touchdown Detection Logic/2(TouchdownFlag) -> Terminator1/1, OR/2  "Pic_TouchdownThreshold"
  CL Based Touchdown Detection Logic/1(EarlyTouchdownFlag) -> Terminator/1, OR/1  "Pic_EarlyTouchdownThreshold"
  FeedbackBus/1 -> Bus Selector/1
  Bus Selector/2 -> Gain/1  "<zAccel_Body_mps2>"
  Bus Selector/3 -> Divide/2  "<DynamicPressure_Pa>"

== system Lib_Piccolo/Ground Detection Systems/WoW Wrapper ==
  note: -1 indicates disarmed. Reverts to using CL touchdown detection
  SimBus : Inport
  FeedbackBus : Inport  Port=2
  Bus Creator : BusCreator  Inputs=6
  Bus Selector : BusSelector  OutputSignals=GrndContactLMG,GrndContactRMG,GrndContactNG,ZgrndLhLbs,ZgrndRhLbs,ZgrndNgLbs
  Bus Selector1 : BusSelector  OutputSignals=ContactBool
  Bus Selector2 : BusSelector  OutputSignals=apMode
  Compare To Constant1 : simulink/Logic and Bit Operations/Compare To Constant  relop=>  const=-1  OutDataTypeStr=uint8
  Constant : Constant  Value=0
  Force Conversion : aerolibconvert2/Force Conversion  IU=lbf  OU=N
      settings: SourceProductName=Aerospace Blockset  SourceProductBaseCode=AE
  Force Conversion1 : aerolibconvert2/Force Conversion  IU=lbf  OU=N
      settings: SourceProductName=Aerospace Blockset  SourceProductBaseCode=AE
  Force Conversion2 : aerolibconvert2/Force Conversion  IU=lbf  OU=N
      settings: SourceProductName=Aerospace Blockset  SourceProductBaseCode=AE
  Pic_WOW_Armed : Constant  Value=WOWarmed
  Switch : Switch  Criteria=u2 > Threshold
  Terminator : Terminator
  Terminator1 : Terminator
  Terminator2 : Terminator
  Variant Subsystem : Subsystem  Variant=on
  TouchdownDetected : Outport
  WoWarmed : Outport  Port=2
  tag scope: Sim_WOWdetect_Signal=global
  wires:
  SimBus/1 -> Bus Selector/1
  Variant Subsystem/1(WOW_Bus_Out) -> Bus Selector1/1
  Bus Selector1/1 -> Switch/1  "<ContactBool>"
  Bus Selector/1 -> Bus Creator/1  "<GrndContactLMG>"
  Bus Selector/2 -> Bus Creator/2  "<GrndContactRMG>"
  Bus Selector/3 -> Bus Creator/3  "<GrndContactNG>"
  Bus Selector/4 -> Bus Creator/4, Force Conversion/1  "<ZgrndLhLbs>"
  Bus Selector/5 -> Bus Creator/5, Force Conversion1/1  "<ZgrndRhLbs>"
  Bus Selector/6 -> Bus Creator/6, Force Conversion2/1  "<ZgrndNgLbs>"
  Bus Creator/1 -> Variant Subsystem/2(WoW_Bus_In)
  Force Conversion/1 -> Terminator/1  "ZgrndLhN"
  Force Conversion1/1 -> Terminator1/1  "ZgrndRhN"
  Force Conversion2/1 -> Terminator2/1  "ZgrndNgN"
  FeedbackBus/1 -> Bus Selector2/1
  Pic_WOW_Armed/1 -> Compare To Constant1/1, WoWarmed/1
  Constant/1 -> Switch/3
  Compare To Constant1/1 -> Switch/2
  Switch/1 -> TouchdownDetected/1, [Sim_WOWdetect_Signal]  "Sim_WOWdetect_Signal"
  Bus Selector2/1 -> Variant Subsystem/1(Piccolo_AP_Mode)  "<apMode>"

== system Lib_Piccolo/Guidance FLIGHT LEGACY/Track Position Decomposition ==
  note: Using dot product to calculate the projection of inertia position & velocity onto the
      | the direction of runway heading and lateral track
  abortFlag : Inport
  TrackHeading_Deg : Inport  Port=2
  VNorth_mps : Inport  Port=3
  VEast_mps : Inport  Port=4
  VDown_mps : Inport  Port=5
  "Xposn_m " : Inport  Port=6
  Yposn_m : Inport  Port=7
  Zposn_m : Inport  Port=8
  Constant{1..4} (4 alike) : Constant  Value=90
  Constant9 : Constant  Value=testPlan(testIndx).Alt
  Cos{1..4} (4 alike) : Trigonometry  Operator=cos
  Cos{5..8} (4 alike) : Trigonometry
  CruiseSlope_Deg : Constant  Value=0
  East : Constant  Value=90
  "East " : Constant  Value=90
  East 1 : Constant  Value=90
  East1 : Constant  Value=90
  Minus{,1..7} (8 alike) : Sum  Inputs=+-
  Multiply{1..8} (8 alike) : Product
  North : Constant  Value=0
  "North " : Constant  Value=0
  North 1 : Constant  Value=0
  North1 : Constant  Value=0
  Saturation : Saturate  UpperLimit=AltMax  LowerLimit=TerrainHeight*0.3048
  Saturation1 : Saturate  UpperLimit=100  LowerLimit=-100
  Sum{1..8} (8 alike) : Sum  Inputs=|++
  Terminator : Terminator
  Terminator1 : Terminator
  deg2rad{1..8} (8 alike) : Gain  Gain=pi/180
  Sim.Ypos : Outport
  "Sim.Vy " : Outport  Port=2
  Sim.Zpos : Outport  Port=3
  Sim.Vz : Outport  Port=4
  Sim.Xpos : Outport  Port=5
  Sim.Vx : Outport  Port=6
  Sim.abortFlag : Outport  Port=7
  wires:
  Cos1/1 -> Multiply7/1
  Yposn_m/1 -> Multiply8/2, Multiply7/2
  Multiply7/1 -> Sum7/2  "EastPosn2LateralPosn"
  Multiply6/1 -> Sum7/1  "NorthPosn2LateralPosn"
  Sum6/1 -> Minus/1, Minus1/1  "Direction of Lateral Track"
  Constant4/1 -> Sum6/2
  Cos3/1 -> Multiply6/1
  "Xposn_m "/1 -> Multiply5/2, Multiply6/2
  Sum7/1 -> Sim.Ypos/1  "Sim.Ypos"
  North/1 -> Minus/2
  Minus/1 -> deg2rad2/1
  Minus1/1 -> deg2rad1/1
  East/1 -> Minus1/2
  deg2rad2/1 -> Cos3/1
  deg2rad1/1 -> Cos1/1
  Sum2/1 -> "Sim.Vy "/1  "Sim.Vy"
  VNorth_mps/1 -> Multiply3/2, Multiply1/2
  Constant1/1 -> Sum1/2
  Cos4/1 -> Multiply1/1
  Multiply2/1 -> Sum2/2  "EastVelocity2LateralVelocity"
  Multiply1/1 -> Sum2/1  "NorthVelocity2LateralVelocity"
  VEast_mps/1 -> Multiply4/2, Multiply2/2
  Minus2/1 -> deg2rad4/1
  "North "/1 -> Minus2/2
  Minus3/1 -> deg2rad3/1
  "East "/1 -> Minus3/2
  deg2rad3/1 -> Cos2/1
  Sum1/1 -> Minus2/1, Minus3/1  "Direction of Lateral Track"
  deg2rad4/1 -> Cos4/1
  Cos2/1 -> Multiply2/1
  Zposn_m/1 -> Terminator1/1
  Minus7/1 -> deg2rad7/1
  Multiply8/1 -> Sum8/2  "EastPosn2LonPosn"
  Cos6/1 -> Multiply4/1
  deg2rad8/1 -> Cos8/1
  deg2rad7/1 -> Cos6/1
  Minus4/1 -> deg2rad6/1
  Minus5/1 -> deg2rad5/1
  Sum3/1 -> Minus6/1, Minus7/1  "Direction of Lon Track"
  TrackHeading_Deg/1 -> Sum6/1, Sum3/1, Sum5/1, Sum1/1
  North 1/1 -> Minus6/2
  Constant3/1 -> Sum5/2
  North1/1 -> Minus4/2
  East1/1 -> Minus5/2
  Constant2/1 -> Sum3/2
  Cos8/1 -> Multiply3/1
  deg2rad5/1 -> Cos5/1
  Sum5/1 -> Minus4/1, Minus5/1  "Direction of Lon Track"
  deg2rad6/1 -> Cos7/1
  Minus6/1 -> deg2rad8/1
  Multiply5/1 -> Sum8/1  "NorthPosn2LonPosn"
  Cos5/1 -> Multiply8/1
  East 1/1 -> Minus7/2
  Multiply3/1 -> Sum4/1  "NorthVelocity2LonVelocity"
  Cos7/1 -> Multiply5/1
  Multiply4/1 -> Sum4/2  "EastVelocity2LonVelocity"
  Sum8/1 -> Sim.Xpos/1  "Sim.Xpos"
  Sum4/1 -> Sim.Vx/1  "Sim.Vx"
  Saturation/1 -> Sim.Zpos/1
  Saturation1/1 -> Sim.Vz/1
  CruiseSlope_Deg/1 -> Saturation1/1
  VDown_mps/1 -> Terminator/1
  abortFlag/1 -> Sim.abortFlag/1
  Constant9/1 -> Saturation/1

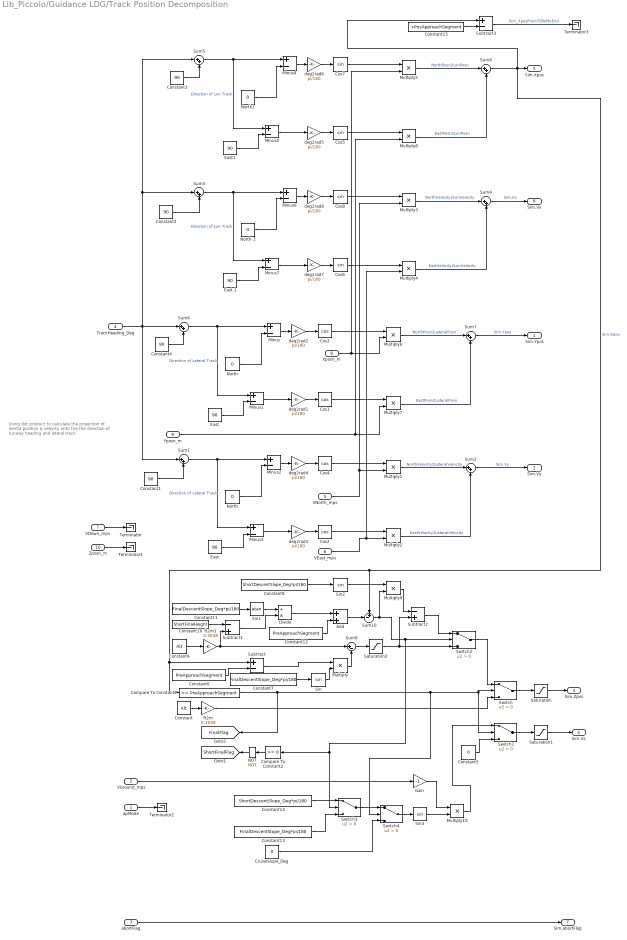
== system Lib_Piccolo/Guidance LDG/Track Position Decomposition ==
  note: Using dot product to calculate the projection of inertia position & velocity onto the
      | the direction of runway heading and lateral track
  apMode : Inport
  VGround_mps : Inport  Port=2
  abortFlag : Inport  Port=3
  TrackHeading_Deg : Inport  Port=4
  VNorth_mps : Inport  Port=5
  VEast_mps : Inport  Port=6
  VDown_mps : Inport  Port=7
  "Xposn_m " : Inport  Port=8
  Yposn_m : Inport  Port=9
  Zposn_m : Inport  Port=10
  Add : Sum
  Compare To Constant1 : simulink/Logic and Bit Operations/Compare To Constant  relop=>=  const=PreApproachSegment  OutDataTypeStr=uint8
  Compare To Constant2 : simulink/Logic and Bit Operations/Compare To Constant  relop=>=  const=0  OutDataTypeStr=uint8
  Constant : Constant  Value=Alt
  Constant{1..4} (4 alike) : Constant  Value=90
  Constant10 : Constant  Value=ShortFinalHeight
  Constant11 : Constant  Value=FinalDescentSlope_Deg*pi/180
  Constant12 : Constant  Value=PreApproachSegment
  Constant13 : Constant  Value=FinalDescentSlope_Deg*pi/180
  Constant14 : Constant  Value=ShortDescentSlope_Deg*pi/180
  Constant15 : Constant  Value=xPosApproachSegment
  Constant5 : Constant  Value=0
  Constant6 : Constant  Value=PreApproachSegment
  Constant7 : Constant  Value=FinalDescentSlope_Deg*pi/180
  Constant8 : Constant  Value=ShortDescentSlope_Deg*pi/180
  Constant9 : Constant  Value=Alt
  Cos{1..4} (4 alike) : Trigonometry  Operator=cos
  Cos{5..8} (4 alike) : Trigonometry
  CruiseSlope_Deg : Constant  Value=0
  Divide : Product  Inputs=/*
  East : Constant  Value=90
  "East " : Constant  Value=90
  East 1 : Constant  Value=90
  East1 : Constant  Value=90
  Gain : Gain  Gain=-1
  Minus{,1..7} (8 alike) : Sum  Inputs=+-
  Multiply{,1..10} (11 alike) : Product
  NOT : Logic  Operator=NOT  IconShape=distinctive  AllPortsSameDT=off  OutDataTypeStr=boolean
  North : Constant  Value=0
  "North " : Constant  Value=0
  North 1 : Constant  Value=0
  North1 : Constant  Value=0
  Saturation : Saturate  UpperLimit=AltMax  LowerLimit=TerrainHeight*0.3048
  Saturation1 : Saturate  UpperLimit=100  LowerLimit=-100
  Saturation2 : Saturate  UpperLimit=AltMax  LowerLimit=ShortFinalHeight
  Sin : Trigonometry
  Sin1 : Trigonometry  Operator=atan
  Sin2 : Trigonometry
  Sin3 : Trigonometry
  Subtract : Sum  Inputs=+-
  Subtract1 : Sum  Inputs=-+
  Subtract2 : Sum  Inputs=-+
  Subtract3 : Sum  Inputs=+-
  Sum{1..8} (8 alike) : Sum  Inputs=|++
  Sum10 : Sum  Inputs=+-|
  Sum9 : Sum  Inputs=|+-
  Switch{,1..4} (5 alike) : Switch  Criteria=u2 > Threshold
  Terminator{,1..3} (4 alike) : Terminator
  deg2rad{1..8} (8 alike) : Gain  Gain=pi/180
  ft2m : Gain  Gain=0.3048
  ft2m1 : Gain  Gain=0.3048
  Sim.Ypos : Outport
  "Sim.Vy " : Outport  Port=2
  Sim.Zpos : Outport  Port=3
  Sim.Vz : Outport  Port=4
  Sim.Xpos : Outport  Port=5
  Sim.Vx : Outport  Port=6
  Sim.abortFlag : Outport  Port=7
  tag scope: FinalFlag=global, ShortFinalFlag=global
  wires:
  Subtract3/1 -> Terminator3/1  "Sim_XposFromTDWPtoEnd"
  Constant15/1 -> Subtract3/2
  Cos1/1 -> Multiply7/1
  Yposn_m/1 -> Multiply8/2, Multiply7/2
  Multiply7/1 -> Sum7/2  "EastPosn2LateralPosn"
  Multiply6/1 -> Sum7/1  "NorthPosn2LateralPosn"
  Sum6/1 -> Minus/1, Minus1/1  "Direction of Lateral Track"
  Constant4/1 -> Sum6/2
  Cos3/1 -> Multiply6/1
  "Xposn_m "/1 -> Multiply5/2, Multiply6/2
  Sum7/1 -> Sim.Ypos/1  "Sim.Ypos"
  North/1 -> Minus/2
  Minus/1 -> deg2rad2/1
  Minus1/1 -> deg2rad1/1
  East/1 -> Minus1/2
  deg2rad2/1 -> Cos3/1
  deg2rad1/1 -> Cos1/1
  Sum2/1 -> "Sim.Vy "/1  "Sim.Vy"
  VNorth_mps/1 -> Multiply3/2, Multiply1/2
  Constant1/1 -> Sum1/2
  Cos4/1 -> Multiply1/1
  Multiply2/1 -> Sum2/2  "EastVelocity2LateralVelocity"
  Multiply1/1 -> Sum2/1  "NorthVelocity2LateralVelocity"
  VEast_mps/1 -> Multiply4/2, Multiply2/2
  Minus2/1 -> deg2rad4/1
  "North "/1 -> Minus2/2
  Minus3/1 -> deg2rad3/1
  "East "/1 -> Minus3/2
  deg2rad3/1 -> Cos2/1
  Sum1/1 -> Minus2/1, Minus3/1  "Direction of Lateral Track"
  deg2rad4/1 -> Cos4/1
  Cos2/1 -> Multiply2/1
  Constant/1 -> ft2m/1
  Zposn_m/1 -> Terminator1/1
  Minus7/1 -> deg2rad7/1
  Multiply8/1 -> Sum8/2  "EastPosn2LonPosn"
  Cos6/1 -> Multiply4/1
  deg2rad8/1 -> Cos8/1
  deg2rad7/1 -> Cos6/1
  Minus4/1 -> deg2rad6/1
  Minus5/1 -> deg2rad5/1
  Sum3/1 -> Minus6/1, Minus7/1  "Direction of Lon Track"
  TrackHeading_Deg/1 -> Sum6/1, Sum3/1, Sum5/1, Sum1/1
  North 1/1 -> Minus6/2
  Constant3/1 -> Sum5/2
  North1/1 -> Minus4/2
  East1/1 -> Minus5/2
  Constant2/1 -> Sum3/2
  Cos8/1 -> Multiply3/1
  deg2rad5/1 -> Cos5/1
  Sum5/1 -> Minus4/1, Minus5/1  "Direction of Lon Track"
  deg2rad6/1 -> Cos7/1
  Minus6/1 -> deg2rad8/1
  Multiply5/1 -> Sum8/1  "NorthPosn2LonPosn"
  Cos5/1 -> Multiply8/1
  East 1/1 -> Minus7/2
  Multiply3/1 -> Sum4/1  "NorthVelocity2LonVelocity"
  Cos7/1 -> Multiply5/1
  Multiply4/1 -> Sum4/2  "EastVelocity2LonVelocity"
  Sum8/1 -> Sum10/1, Compare To Constant1/1, Subtract/1, Sim.Xpos/1, Subtract3/1  "Sim.Xpos"
  Sum4/1 -> Sim.Vx/1  "Sim.Vx"
  Saturation/1 -> Sim.Zpos/1
  ft2m/1 -> Switch/3
  Constant5/1 -> Switch1/3
  Saturation1/1 -> Sim.Vz/1
  Switch1/1 -> Saturation1/1
  Switch/1 -> Saturation/1
  Constant6/1 -> Subtract/2
  Constant7/1 -> Sin/1
  Subtract/1 -> Multiply/1
  Sin/1 -> Multiply/2
  Constant9/1 -> ft2m1/1
  ft2m1/1 -> Subtract1/2, Sum9/1
  Multiply/1 -> Sum9/2
  Sum9/1 -> Saturation2/1
  Constant10/1 -> Subtract1/1
  Constant11/1 -> Sin1/1
  Sin1/1 -> Divide/1
  Subtract1/1 -> Divide/2
  VDown_mps/1 -> Terminator/1
  Divide/1 -> Add/1
  Constant12/1 -> Add/2
  Add/1 -> Sum10/2
  Saturation2/1 -> Subtract2/2, Switch2/3
  Constant8/1 -> Sin2/1
  Sin2/1 -> Multiply9/1
  Sum10/1 -> Switch3/2, Compare To Constant2/1, Switch2/2, Multiply9/2
  Multiply9/1 -> Subtract2/1
  Subtract2/1 -> Switch2/1
  Switch2/1 -> Switch/1
  Switch3/1 -> Switch4/1
  CruiseSlope_Deg/1 -> Switch4/3
  Switch4/1 -> Sin3/1
  VGround_mps/1 -> Gain/1
  Sin3/1 -> Multiply10/2
  Gain/1 -> Multiply10/1
  Multiply10/1 -> Switch1/1
  Constant14/1 -> Switch3/1
  Constant13/1 -> Switch3/3
  apMode/1 -> Terminator2/1
  Compare To Constant2/1 -> NOT/1
  NOT/1 -> [ShortFinalFlag]
  abortFlag/1 -> Sim.abortFlag/1
  Compare To Constant1/1 -> Switch4/2, Switch/2, Switch1/2, [FinalFlag]

== system Lib_Piccolo/Guidance Takeoff & Flight/Track Position Decomposition ==
  apMode : Inport
  VGround_mps : Inport  Port=2
  abortFlag : Inport  Port=3
  TrackHeading_Deg : Inport  Port=4
  VNorth_mps : Inport  Port=5
  VEast_mps : Inport  Port=6
  VDown_mps : Inport  Port=7
  "Xposn_m " : Inport  Port=8
  Yposn_m : Inport  Port=9
  Zposn_m : Inport  Port=10
  Flight Guidance : Subsystem
  Landing Guidance : Subsystem
  Terminator{,1..8} (9 alike) : Terminator
  Sim.Ypos : Outport
  "Sim.Vy " : Outport  Port=2
  Sim.Zpos : Outport  Port=3
  Sim.Vz : Outport  Port=4
  Sim.Xpos : Outport  Port=5
  Sim.Vx : Outport  Port=6
  Sim.abortFlag : Outport  Port=7
  wires:
  Zposn_m/1 -> Terminator1/1
  VDown_mps/1 -> Terminator/1
  apMode/1 -> Terminator2/1
  abortFlag/1 -> Sim.abortFlag/1
  TrackHeading_Deg/1 -> Landing Guidance/1(TrackHeading_Deg), Flight Guidance/1(TrackHeading_Deg)  "TrackHeading_Deg"
  "Xposn_m "/1 -> Landing Guidance/2(Xposn_m), Flight Guidance/2(Xposn_m)  "Xposn_m"
  Yposn_m/1 -> Landing Guidance/3(Yposn_m), Flight Guidance/3(Yposn_m)  "Yposn_m"
  VNorth_mps/1 -> Landing Guidance/4(VNorth_mps), Flight Guidance/4(VNorth_mps)
  VEast_mps/1 -> Landing Guidance/5(VEast_mps), Flight Guidance/5(VEast_mps)
  VGround_mps/1 -> Landing Guidance/6(VGround_mps), Flight Guidance/6(VGround_mps)  "VGround_mps"
  Flight Guidance/1(Sim.Xpos) -> Sim.Xpos/1
  Flight Guidance/2(Sim.Vx) -> Sim.Vx/1
  Flight Guidance/3(Sim.Ypos) -> Sim.Ypos/1
  Flight Guidance/4(Sim.Vy) -> "Sim.Vy "/1
  Flight Guidance/5(Sim.Zpos) -> Sim.Zpos/1
  Flight Guidance/6(Sim.Vz) -> Sim.Vz/1
  Landing Guidance/1(Sim.Xpos) -> Terminator3/1
  Landing Guidance/2(Sim.Vx) -> Terminator4/1
  Landing Guidance/3(Sim.Ypos) -> Terminator5/1
  Landing Guidance/4(Sim.Vy) -> Terminator6/1
  Landing Guidance/5(Sim.Zpos) -> Terminator7/1
  Landing Guidance/6(Sim.Vz) -> Terminator8/1

== system Lib_Piccolo/Heading Control/LPF Heading ==
  Input : Inport
  Reset : Inport  Port=2
  Add1 : Sum  Inputs=++|
  Compare To Constant2 : simulink/Logic and Bit Operations/Compare To Constant  relop=>  const=0  OutDataTypeStr=uint8
  Constant11 : Constant  Value=TurnErrLPFcutoff
  Switch1 : Switch  Criteria=u2 > Threshold
  Unit Delay1 : UnitDelay  InitialCondition=LPFturnErrInit  SampleTime=-1
  a1 : Gain  Gain=1-Fp_Turn
  b0 : Gain  Gain=Fp_Turn
  Output : Outport
  wires:
  Constant11/1 -> Compare To Constant2/1
  Compare To Constant2/1 -> Switch1/2
  Switch1/1 -> Output/1
  Input/1 -> b0/1, Switch1/3
  Add1/1 -> Switch1/1, Unit Delay1/1
  a1/1 -> Add1/1
  b0/1 -> Add1/2
  Unit Delay1/1 -> a1/1

== system Lib_Piccolo/Heading Control/LPF HeadingDerivative ==
  Input : Inport
  Reset : Inport  Port=2
  Add1 : Sum  Inputs=++|
  Compare To Constant2 : simulink/Logic and Bit Operations/Compare To Constant  relop=>  const=0  OutDataTypeStr=uint8
  Constant11 : Constant  Value=TurnDerivativeLPFcutoff
  Switch1 : Switch  Criteria=u2 > Threshold
  Unit Delay1 : UnitDelay  SampleTime=-1
  a1 : Gain  Gain=1-Fp_TurnDerr
  b0 : Gain  Gain=Fp_TurnDerr
  Output : Outport
  wires:
  Constant11/1 -> Compare To Constant2/1
  Compare To Constant2/1 -> Switch1/2
  Switch1/1 -> Output/1
  Input/1 -> b0/1, Switch1/3
  Add1/1 -> Switch1/1, Unit Delay1/1
  a1/1 -> Add1/1
  b0/1 -> Add1/2
  Unit Delay1/1 -> a1/1

== system Lib_Piccolo/Heading Control/On Ground ==
  GuidanceBankCmd : Inport
  <apMode> : Inport  Port=2
  Compare To Constant1 : simulink/Logic and Bit Operations/Compare To Constant  relop=<=  const=1  OutDataTypeStr=uint8
  Compare To Constant2 : simulink/Logic and Bit Operations/Compare To Constant  relop===  const=11  OutDataTypeStr=uint8
  GroundBankCmd : Constant  Value=0
  OR : Logic  Operator=OR  IconShape=distinctive  AllPortsSameDT=off  OutDataTypeStr=boolean
  Switch : Switch  Criteria=u2 > Threshold
  BankCmd : Outport
  wires:
  Compare To Constant2/1 -> OR/1
  <apMode>/1 -> Compare To Constant1/1, Compare To Constant2/1
  GroundBankCmd/1 -> Switch/1
  GuidanceBankCmd/1 -> Switch/3
  Switch/1 -> BankCmd/1
  OR/1 -> Switch/2
  Compare To Constant1/1 -> OR/2

== system Lib_Piccolo/Heading Control/UnwindHdg ==
  REF.yaw : Inport
  Compare To Constant3 : simulink/Logic and Bit Operations/Compare To Constant  relop=>  const=180  OutDataTypeStr=boolean
  Constant : Constant  Value=360
  Subtract : Sum  Inputs=+-
  Switch : Switch  Criteria=u2 > Threshold
  Out1 : Outport
  wires:
  REF.yaw/1 -> Subtract/1, Compare To Constant3/1, Switch/3
  Compare To Constant3/1 -> Switch/2
  Switch/1 -> Out1/1
  Constant/1 -> Subtract/2
  Subtract/1 -> Switch/1

== system Lib_Piccolo/Heading Control/UnwindHdg1 ==
  REF.yaw : Inport
  Compare To Constant3 : simulink/Logic and Bit Operations/Compare To Constant  relop=>  const=180  OutDataTypeStr=boolean
  Constant : Constant  Value=360
  Subtract : Sum  Inputs=+-
  Switch : Switch  Criteria=u2 > Threshold
  Out1 : Outport
  wires:
  REF.yaw/1 -> Subtract/1, Compare To Constant3/1, Switch/3
  Compare To Constant3/1 -> Switch/2
  Switch/1 -> Out1/1
  Constant/1 -> Subtract/2
  Subtract/1 -> Switch/1

== system Lib_Piccolo/Heading Control/WindCorrectionEstimate ==
  WindSouth : Inport
  WindWest : Inport  Port=2
  Rad2Deg : Gain  Gain=180/pi
  Sqrt : Sqrt  SaturateOnIntegerOverflow=on
  Square : Math  Operator=square  SaturateOnIntegerOverflow=on
  Square1 : Math  Operator=square  SaturateOnIntegerOverflow=on
  Subtract : Sum
  Trigonometric Function2 : Trigonometry  Operator=atan2
  WindMag : Outport
  WindDir : Outport  Port=2
  wires:
  WindSouth/1 -> Square/1, Trigonometric Function2/2
  Square/1 -> Subtract/1
  Square1/1 -> Subtract/2
  Subtract/1 -> Sqrt/1
  Sqrt/1 -> WindMag/1  "Sim.WindMagnitude"
  WindWest/1 -> Square1/1, Trigonometric Function2/1
  Trigonometric Function2/1 -> Rad2Deg/1
  Rad2Deg/1 -> WindDir/1  "Sim.WindDirection"

== system Lib_Piccolo/LDG TAS Cmd/CAS2TAS ==
  In1 : Inport
  Bus Selector2 : BusSelector  OutputSignals=airDensity_kgm
  Constant : Constant  Value=1.225
  Divide : Product  Inputs=*/
  Sqrt : Sqrt  SaturateOnIntegerOverflow=on
  Out1 : Outport
  wires:
  In1/1 -> Bus Selector2/1
  Bus Selector2/1 -> Divide/2  "<airDensity_kgm>"
  Constant/1 -> Divide/1
  Divide/1 -> Sqrt/1
  Sqrt/1 -> Out1/1

== system Lib_Piccolo/LDG TAS Cmd No Offset/CAS2TAS ==
  In1 : Inport
  Bus Selector2 : BusSelector  OutputSignals=airDensity_kgm
  Constant : Constant  Value=1.225
  Divide : Product  Inputs=*/
  Sqrt : Sqrt  SaturateOnIntegerOverflow=on
  Out1 : Outport
  wires:
  In1/1 -> Bus Selector2/1
  Bus Selector2/1 -> Divide/2  "<airDensity_kgm>"
  Constant/1 -> Divide/1
  Divide/1 -> Sqrt/1
  Sqrt/1 -> Out1/1
